simulink model "MMC_driven_PMSM_ideal"  (R2025b)
settings: Solver=FixedStepDiscrete  StartTime=0.0  StopTime=7  FixedStep=Ts  RelTol=1e-3
values from neighbouring files (symbols this model uses):
  Goff = 1e-06    [initParams.mat]
  Ron = 1e-06    [initParams.mat]
  Ts = 5e-05    [initParams.mat]
  Vcell = 1000    [initParams.mat]
undefined symbols (not defined in the file or in its folder): DiscIntNeverNeededParam
libraries: ee_lib_for_power_systems x50, fl_lib x48, nesl_utility x3, eeTransforms x2, ee_lib x2, simulink x1
(part 1 of 2)
settings Model: SimulationMode=accelerator  Creator=gdudgeon  LastModifiedBy=gdudgeon
settings SolverCC: AlgebraicLoopSolver=TrustRegion
settings DebuggingCC: UnconnectedInputMsg=warning  UnconnectedOutputMsg=warning  UnconnectedLineMsg=warning
settings ModelReferenceCC: EnableRefExpFcnMdlSchedulingChecks=on
settings RTWCC: GPUComputeCapability=3.5

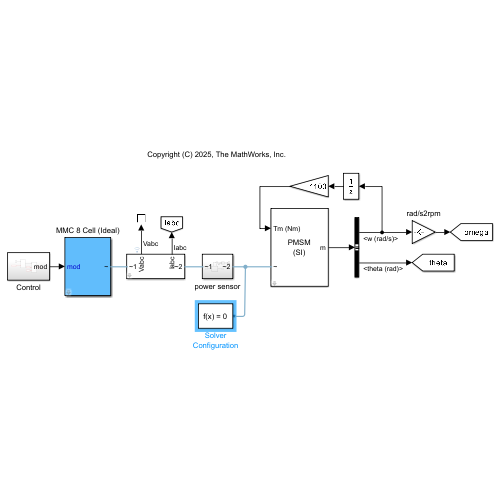
[thumbnail: Simulink's stored preview of the top-level diagram]
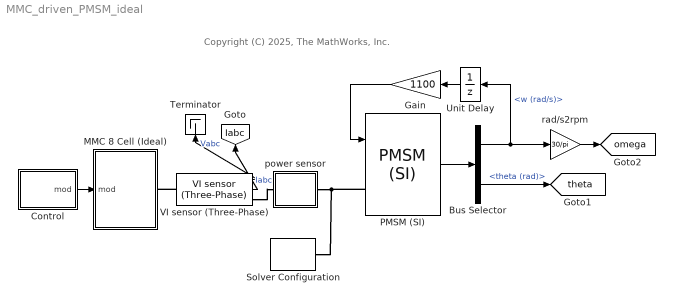
== system MMC_driven_PMSM_ideal ==
  note: Copyright (C) 2025, The MathWorks, Inc.
  Bus Selector : BusSelector  OutputSignals=w (rad/s),theta (rad)
  Control : Subsystem
  Gain : Gain  Gain=1100
  MMC 8 Cell (Ideal) : Subsystem  mask{Vcell=Vcell, freq=1000, no_cells=8}
      mask prompts: Vcell "Cell voltage (V)"; freq "Carrier frequency (Hz)"; no_cells "Number of cells"
  PMSM (SI) : ee_lib_for_power_systems/Electromechanical Machines/PMSM (SI)  run_time=on  p=1  flux_linkage=21  Ld=0.0005  Lq=0.0005  Rs=0.01  J=10  D=0
      settings: SourceProductName=Support Library for Power Systems
  Solver Configuration : nesl_utility/Solver Configuration  PhysicalDomain=network_engine_domain  SubClassName=solver  LeftPortType=input  RightPortType=generic  Tones=[]  Harmonics=[]  SimulateNoise=off  Profile=off  UseLocalSampling=off  EnableSwitchedLinearOptims=on  FrequencyDomain=off  UseCCode=off  RelTol=0.001  AbsTol=1e-06  MinStep=1e-09  ToWorkspace=off  RevertToSquareIcSolve=off  NumHomotopyIterations=100  PhasorMode=off  PhasorModeNumHarmonics=1  ConsistencySolver=NEWTON_FTOL  IndexReductionMethod=None  DoDC=off  ResidualTolerance=1e-09  ConsistencyTolSource=GLOBAL  ConsistencyAbsTol=0.001  ConsistencyRelTol=0.001  ConsistencyTolFactor=0.001  UseLocalSolver=on  LocalSolverChoice=NE_BACKWARD_EULER_ADVANCER  ResolveIndetEquations=off  FunctionEvalNumThread=1  LocalSolverSampleTime=TsELEC  DoFixedCost=on  MaxNonlinIter=1  MaxModeIter=2  ComputeImpulses=off  ImpulseIterations=2  LinearAlgebra=auto  LinearAlgebraNumThread=0  EquationFormulation=NE_TIME_EF  DelaysMemoryBudget=1024  AutomaticFiltering=off  FilteringTimeConstant=0.001  PartitionStorageMethod=AS_NEEDED  PartitionMemoryBudget=1024  PartitionMethod=ROBUST  MultibodyUseLocalSolver=off  MultibodyLocalSolverChoice=ODE1  MultibodyLocalSolverSampleTime=0.001
  Terminator : Terminator
  Unit Delay : UnitDelay  SampleTime=-1  HasFrameUpgradeWarning=on
  VI sensor (Three-Phase) : ee_lib_for_power_systems/Sense and Measure/VI sensor (Three-Phase)  volt_meas=Line-to-Line (Line Voltage)  meas_units=SI  Vnom=24e3  Pnom=100e6
      settings: SourceProductName=Support Library for Power Systems
  power sensor : Subsystem
  rad/s2rpm : Gain  Gain=30/pi
  tag scope: Iabc=global, omega=global, theta=global
  wires:
  Control/1(mod) -> MMC 8 Cell (Ideal)/1(mod)
  VI sensor (Three-Phase)/1 -> Terminator/1  "Vabc"
  VI sensor (Three-Phase)/2 -> [Iabc]  "Iabc"
  PMSM (SI)/1 -> Bus Selector/1
  Bus Selector/2 -> [theta]  "<theta (rad)>"
  Bus Selector/1 -> Unit Delay/1, rad/s2rpm/1  "<w (rad/s)>"
  Gain/1 -> PMSM (SI)/1
  Unit Delay/1 -> Gain/1
  rad/s2rpm/1 -> [omega]
  connections:
  VI sensor (Three-Phase)/RConn1 -- power sensor/LConn1
  VI sensor (Three-Phase)/LConn1 -- MMC 8 Cell (Ideal)/RConn1
  power sensor/RConn1 -- PMSM (SI)/LConn1 -- Solver Configuration/RConn1

== system MMC_driven_PMSM_ideal/Control ==
  Dead Zone : DeadZone  LowerValue=-0.001  UpperValue=0.001
  Speed Control : Subsystem
  Speed Reference (RPM) : simulink/Sources/Repeating Sequence Interpolated  OutValues=[0 0 1 1]*1800  TimeValues=[0 1 6 15]  LookUpMeth=Interpolation-Use End Values  tsamp=TsELEC  OutMin=[]  OutMax=[]  OutDataTypeStr=double  OutputDataTypeScalingMode=double  OutDataType=fixdt(0,8)  OutScaling=2^-10
  Torque Control : Subsystem
  Unit Delay1 : UnitDelay  SampleTime=Ts  HasFrameUpgradeWarning=on
  mod : Outport
  wires:
  Unit Delay1/1 -> Dead Zone/1
  Speed Reference (RPM)/1 -> Speed Control/1(Speed_Ref)  "omega_ref"
  Torque Control/1(mod) -> Unit Delay1/1
  [omega] -> Speed Control/2(Speed_Meas)  "omega"
  Speed Control/1(IdqRef) -> Torque Control/1(Idq_ref)
  [Iabc] -> Torque Control/2(Iabc_meas)
  [theta] -> Torque Control/3(theta)
  Dead Zone/1 -> mod/1

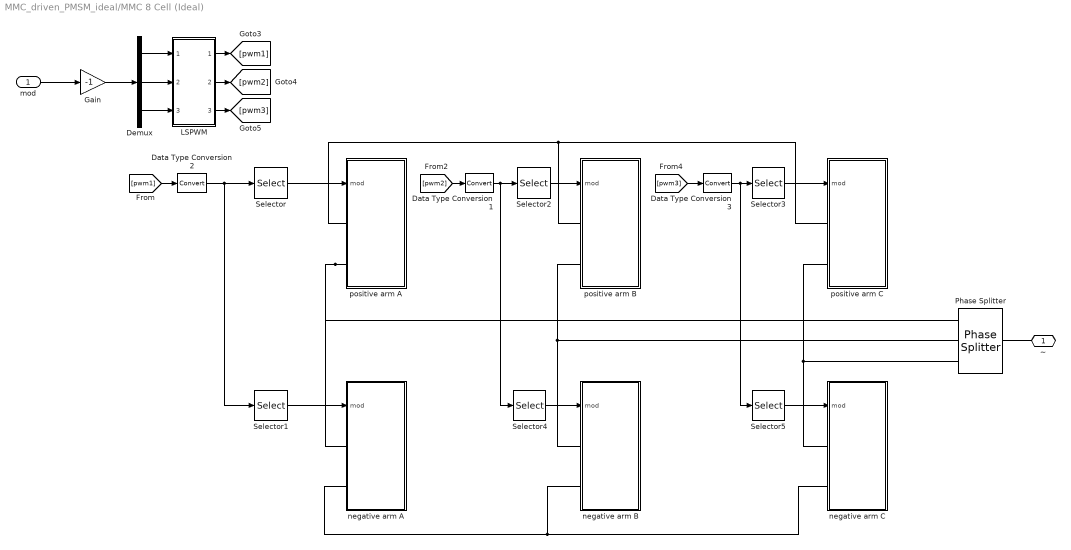
== system MMC_driven_PMSM_ideal/MMC 8 Cell (Ideal) ==
  mod : Inport
  Data Type Conversion1 : DataTypeConversion  SaturateOnIntegerOverflow=off  RndMeth=Floor
  Data Type Conversion2 : DataTypeConversion  SaturateOnIntegerOverflow=off  RndMeth=Floor
  Data Type Conversion3 : DataTypeConversion  SaturateOnIntegerOverflow=off  RndMeth=Floor
  Demux : Demux  Outputs=3
  Gain : Gain  Gain=-1
  LSPWM : Subsystem  mask{no_cells=no_cells, freq=freq}
      mask prompts: no_cells "Number of cells"; freq "Carrier frequency (Hz)"
  Phase Splitter : ee_lib/Connectors & References/Phase Splitter
  Selector : Selector  InputPortWidth=no_cells*4  IndexOptions=Index vector (dialog)  Indices=[1:(no_cells) (no_cells*2+1):no_cells*3]  OutputSizes=1
  Selector1 : Selector  InputPortWidth=no_cells*4  IndexOptions=Index vector (dialog)  Indices=[(no_cells)+(1:no_cells) (no_cells*3)+(1:no_cells)]  OutputSizes=1
  Selector2 : Selector  InputPortWidth=no_cells*4  IndexOptions=Index vector (dialog)  Indices=[1:(no_cells) (no_cells*2+1):no_cells*3]  OutputSizes=1
  Selector3 : Selector  InputPortWidth=no_cells*4  IndexOptions=Index vector (dialog)  Indices=[1:(no_cells) (no_cells*2+1):no_cells*3]  OutputSizes=1
  Selector4 : Selector  InputPortWidth=no_cells*4  IndexOptions=Index vector (dialog)  Indices=[(no_cells)+(1:no_cells) (no_cells*3)+(1:no_cells)]  OutputSizes=1
  Selector5 : Selector  InputPortWidth=no_cells*4  IndexOptions=Index vector (dialog)  Indices=[(no_cells)+(1:no_cells) (no_cells*3)+(1:no_cells)]  OutputSizes=1
  negative arm A : Subsystem  mask{Vcell=Vcell, no_cells=no_cells, Ron=Ron, Goff=Goff}
      mask prompts: Vcell "Cell Voltage (V)"; no_cells "Number of cells"; Ron "Ron (Ohm)"; Goff "Goff (1/Ohm)"
      mask init:
      | h = gcbh;
      | 
      | hr = find_system(h,'LookUnderMasks','All','RegExp','on','Name','rmod');
      | hs = find_system(h,'LookUnderMasks','All','RegExp','on','Name','smod');
      | 
      | for l = 1:numel(hr)
      |     
      |     nr = get(hr(l),'name');
      |     ns = get(hs(l),'name');
      |     
      |     set(hr(l),'GotoTag',nr(2:end));
      |     set(hs(l),'GotoTag',nr(2:end));
      |     
      | end
      |     
      | rr = zeros(1,no_cells*2);
      | rr(1:2:end) = 1:no_cells;
      | rr(2:2:end) = (no_cells+1):2*no_cells;
  negative arm B : Subsystem  mask{Vcell=Vcell, no_cells=no_cells, Ron=Ron, Goff=Goff}
      mask prompts: Vcell "Cell Voltage (V)"; no_cells "Number of cells"; Ron "Ron (Ohm)"; Goff "Goff (1/Ohm)"
      mask init: same as MMC_driven_PMSM_ideal/MMC 8 Cell (Ideal)/negative arm A
  negative arm C : Subsystem  mask{Vcell=Vcell, no_cells=no_cells, Ron=Ron, Goff=Goff}
      mask prompts: Vcell "Cell Voltage (V)"; no_cells "Number of cells"; Ron "Ron (Ohm)"; Goff "Goff (1/Ohm)"
      mask init: same as MMC_driven_PMSM_ideal/MMC 8 Cell (Ideal)/negative arm A
  positive arm A : Subsystem  mask{Vcell=Vcell, no_cells=no_cells, Ron=Ron, Goff=Goff}
      mask prompts: Vcell "Cell Voltage (V)"; no_cells "Number of cells"; Ron "Ron (Ohm)"; Goff "Goff (1/Ohm)"
      mask init: same as MMC_driven_PMSM_ideal/MMC 8 Cell (Ideal)/negative arm A
  positive arm B : Subsystem  mask{Vcell=Vcell, no_cells=no_cells, Ron=Ron, Goff=Goff}
      mask prompts: Vcell "Cell Voltage (V)"; no_cells "Number of cells"; Ron "Ron (Ohm)"; Goff "Goff (1/Ohm)"
      mask init: same as MMC_driven_PMSM_ideal/MMC 8 Cell (Ideal)/negative arm A
  positive arm C : Subsystem  mask{Vcell=Vcell, no_cells=no_cells, Ron=Ron, Goff=Goff}
      mask prompts: Vcell "Cell Voltage (V)"; no_cells "Number of cells"; Ron "Ron (Ohm)"; Goff "Goff (1/Ohm)"
      mask init: same as MMC_driven_PMSM_ideal/MMC 8 Cell (Ideal)/negative arm A
  ~ : PMIOPort  Side=Right
  wires:
  Gain/1 -> Demux/1
  Selector5/1 -> negative arm C/1(mod)
  Selector3/1 -> positive arm C/1(mod)
  Selector4/1 -> negative arm B/1(mod)
  Selector2/1 -> positive arm B/1(mod)
  Selector/1 -> positive arm A/1(mod)
  LSPWM/3("      ") -> [pwm3]
  LSPWM/2("       ") -> [pwm2]
  LSPWM/1(" ") -> [pwm1]
  [pwm3] -> Data Type Conversion3/1
  [pwm2] -> Data Type Conversion1/1
  [pwm1] -> Data Type Conversion2/1
  Demux/3 -> LSPWM/3("     ")
  Demux/2 -> LSPWM/2("   ")
  Demux/1 -> LSPWM/1("  ")
  mod/1 -> Gain/1
  Data Type Conversion2/1 -> Selector1/1, Selector/1
  Data Type Conversion3/1 -> Selector5/1, Selector3/1
  Data Type Conversion1/1 -> Selector2/1, Selector4/1
  Selector1/1 -> negative arm A/1(mod)
  connections:
  Phase Splitter/RConn2 -- negative arm B/LConn1 -- positive arm B/LConn2
  positive arm A/LConn2 -- negative arm A/LConn1 -- Phase Splitter/RConn1
  Phase Splitter/RConn3 -- positive arm C/LConn2 -- negative arm C/LConn1
  positive arm A/LConn1 -- positive arm C/LConn1 -- positive arm B/LConn1
  negative arm A/LConn2 -- negative arm C/LConn2 -- negative arm B/LConn2
  ~/RConn1 -- Phase Splitter/LConn1

== system MMC_driven_PMSM_ideal/power sensor ==
  PS-Simulink Converter : nesl_utility/PS-Simulink Converter  PhysicalDomain=network_engine_domain  SubClassName=ps_output  LeftPortType=input  RightPortType=output  PseudoPeriodic=off  Frequencies=[]  VectorFormat=inherit  Unit=inherit  AffineConversion=off
  PS-Simulink Converter1 : nesl_utility/PS-Simulink Converter  PhysicalDomain=network_engine_domain  SubClassName=ps_output  LeftPortType=input  RightPortType=output  PseudoPeriodic=off  Frequencies=[]  VectorFormat=inherit  Unit=inherit  AffineConversion=off
  Power Sensor (Three-Phase) : ee_lib/Sensors & Transducers/Power Sensor (Three-Phase)  load_type=ee.enum.passive.type_balanced.balanced  f0=60 Hz
      settings: InternalSimscapePortConfiguration="{\"Bottom\":[],\"Left\":[{\"id\":\"N1\",\"label\":\"~1\",\"type\":\"foundation.electrical.three_phase\"}],\"Right\":[{\"id\":\"N2\",\"label\":\"~2\",\"type\":\"foundation.electrical.three_phase\"}],\"Top\":[{\"id\":\"Pm\",\"label\":\"P\",\"type\":\"output\"},{\"id\":\"Qm\",\"label\":\"Q\",\"type\":\"output\"}]}"
  Subsystem1 : Subsystem
  Subsystem2 : Subsystem
  Terminator : Terminator
  Terminator1 : Terminator
  ~1 : PMIOPort  Side=Left
  ~2 : PMIOPort  Port=2  Side=Right
  wires:
  PS-Simulink Converter/1 -> Subsystem1/1(In1)
  PS-Simulink Converter1/1 -> Subsystem2/1(In1)
  Subsystem2/1(Out1) -> Terminator1/1  "Q"
  Subsystem1/1(Out1) -> Terminator/1  "P"
  connections:
  Power Sensor (Three-Phase)/LConn2 -- PS-Simulink Converter/LConn1
  Power Sensor (Three-Phase)/RConn1 -- ~2/RConn1
  Power Sensor (Three-Phase)/LConn1 -- ~1/RConn1
  Power Sensor (Three-Phase)/LConn3 -- PS-Simulink Converter1/LConn1

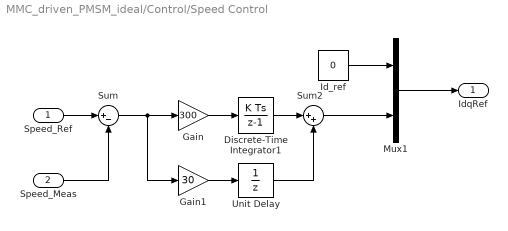
== system MMC_driven_PMSM_ideal/Control/Speed Control ==
  Speed_Ref : Inport
  Speed_Meas : Inport  Port=2
  Discrete-Time Integrator1 : DiscreteIntegrator  SampleTime=Ts  ICPrevOutput=DiscIntNeverNeededParam  ICPrevScaledInput=DiscIntNeverNeededParam
  Gain : Gain  Gain=300
  Gain1 : Gain  Gain=30
  Id_ref : Constant  Value=0  OutDataTypeStr=Inherit: Inherit via back propagation  SampleTime=Ts
  Mux1 : Mux  Inputs=2
  Sum : Sum  Inputs=|+-
  Sum2 : Sum  Inputs=|++
  Unit Delay : UnitDelay  SampleTime=Ts  HasFrameUpgradeWarning=on
  IdqRef : Outport  VectorParamsAs1DForOutWhenUnconnected=off
  wires:
  Sum2/1 -> Mux1/2
  Id_ref/1 -> Mux1/1
  Speed_Ref/1 -> Sum/1
  Speed_Meas/1 -> Sum/2
  Mux1/1 -> IdqRef/1
  Gain/1 -> Discrete-Time Integrator1/1
  Sum/1 -> Gain1/1, Gain/1
  Unit Delay/1 -> Sum2/2
  Gain1/1 -> Unit Delay/1
  Discrete-Time Integrator1/1 -> Sum2/1

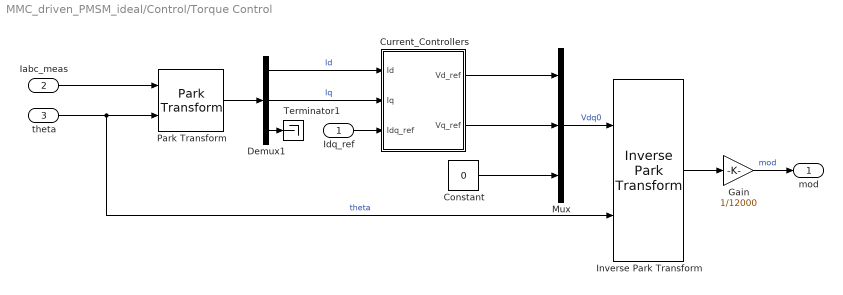
== system MMC_driven_PMSM_ideal/Control/Torque Control ==
  Idq_ref : Inport
  Iabc_meas : Inport  Port=2
  theta : Inport  Port=3
  Constant : Constant  Value=0  SampleTime=Ts
  Current_Controllers : Subsystem
  Demux1 : Demux  Outputs=3
  Gain : Gain  Gain=1/12000
  Inverse Park Transform : eeTransforms/Inverse Park Transform  AxisAlignment=Q-axis  PowerInvariant=off
  Mux : Mux  Inputs=3
  Park Transform : eeTransforms/Park Transform  AxisAlignment=Q-axis  PowerInvariant=off
      settings: LibrarySourceBlock=|
      | ee_sl_lib/Mathematical
      | Transforms/Park Transform
  Terminator1 : Terminator
  mod : Outport  VectorParamsAs1DForOutWhenUnconnected=off
  wires:
  Current_Controllers/1(Vd_ref) -> Mux/1
  Gain/1 -> mod/1  "mod"
  Idq_ref/1 -> Current_Controllers/3(Idq_ref)
  Inverse Park Transform/1 -> Gain/1
  Park Transform/1 -> Demux1/1
  Constant/1 -> Mux/3
  Demux1/2 -> Current_Controllers/2(Iq)  "Iq"
  Current_Controllers/2(Vq_ref) -> Mux/2
  Demux1/3 -> Terminator1/1
  Mux/1 -> Inverse Park Transform/1  "Vdq0"
  theta/1 -> Inverse Park Transform/2, Park Transform/2  "theta"
  Demux1/1 -> Current_Controllers/1(Id)  "Id"
  Iabc_meas/1 -> Park Transform/1

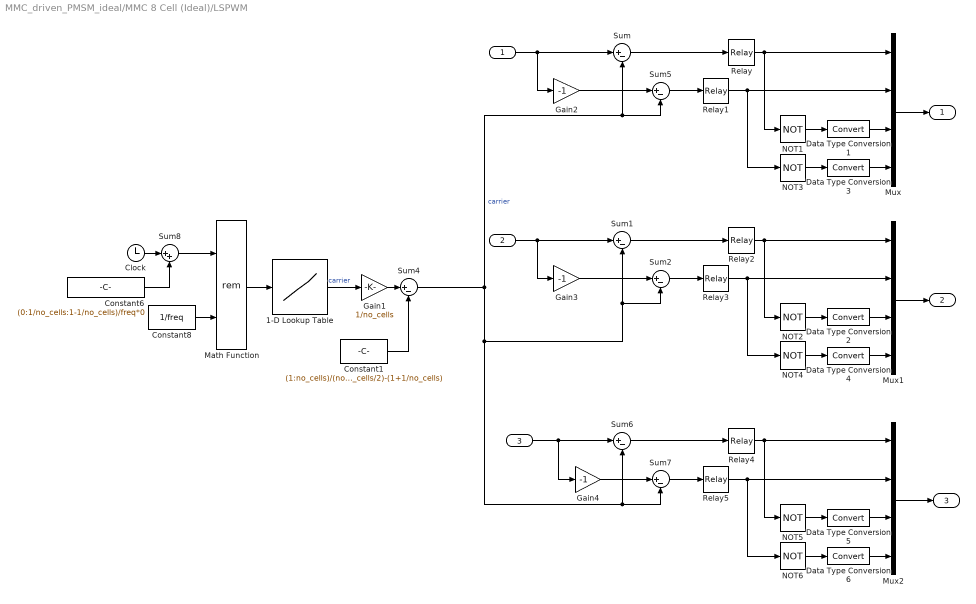
== system MMC_driven_PMSM_ideal/MMC 8 Cell (Ideal)/LSPWM ==
  "  " : Inport
  "   " : Inport  Port=2
  "     " : Inport  Port=3
  1-D Lookup Table : Lookup_n-D  NumberOfTableDimensions=1  BreakpointsForDimension1=[0 1 2 3 4]/4/freq  Table=[0 1 0 -1 0]  RndMeth=Simplest
  Clock : Clock
  Constant1 : Constant  DisableCoverage=on  Value=(1:no_cells)/(no_cells/2)-(1+1/no_cells)  SampleTime=0
  Constant6 : Constant  Value=(0:1/no_cells:1-1/no_cells)/freq*0  SampleTime=0
  Constant8 : Constant  DisableCoverage=on  Value=1/freq  SampleTime=0
  Data Type Conversion{1..6} (6 alike) : DataTypeConversion  SaturateOnIntegerOverflow=off  RndMeth=Floor
  Gain1 : Gain  Gain=1/no_cells
  Gain2 : Gain  Gain=-1
  Gain3 : Gain  Gain=-1
  Gain4 : Gain  Gain=-1
  Math Function : Math  DisableCoverage=on  Operator=rem  SignedPower=on
  Mux : Mux
  Mux1 : Mux
  Mux2 : Mux
  NOT{1..6} (6 alike) : Logic  Operator=NOT  IconShape=distinctive  AllPortsSameDT=off  OutDataTypeStr=boolean
  Relay{,1..5} (6 alike) : Relay
  Sum{,1..2,4..7} (7 alike) : Sum  Inputs=|+-
  Sum8 : Sum  Inputs=|++
  " " : Outport  VectorParamsAs1DForOutWhenUnconnected=off
  "       " : Outport  Port=2  VectorParamsAs1DForOutWhenUnconnected=off
  "      " : Outport  Port=3  VectorParamsAs1DForOutWhenUnconnected=off
  wires:
  Sum4/1 -> Sum/2, Sum5/2, Sum6/2, Sum7/2, Sum2/2, Sum1/2  "carrier"
  Relay5/1 -> Mux2/2, NOT6/1
  Sum7/1 -> Relay5/1
  Gain4/1 -> Sum7/1
  Data Type Conversion6/1 -> Mux2/4
  NOT6/1 -> Data Type Conversion6/1
  Data Type Conversion5/1 -> Mux2/3
  "     "/1 -> Gain4/1, Sum6/1
  Sum6/1 -> Relay4/1
  Relay4/1 -> Mux2/1, NOT5/1
  NOT5/1 -> Data Type Conversion5/1
  Mux2/1 -> "      "/1
  Mux1/1 -> "       "/1
  NOT2/1 -> Data Type Conversion2/1
  Relay2/1 -> NOT2/1, Mux1/1
  Sum1/1 -> Relay2/1
  "   "/1 -> Sum1/1, Gain3/1
  Data Type Conversion2/1 -> Mux1/3
  NOT4/1 -> Data Type Conversion4/1
  Data Type Conversion4/1 -> Mux1/4
  Gain3/1 -> Sum2/1
  Sum2/1 -> Relay3/1
  Relay3/1 -> NOT4/1, Mux1/2
  Relay1/1 -> Mux/2, NOT3/1
  Sum5/1 -> Relay1/1
  Gain2/1 -> Sum5/1
  Data Type Conversion3/1 -> Mux/4
  NOT3/1 -> Data Type Conversion3/1
  Data Type Conversion1/1 -> Mux/3
  Gain1/1 -> Sum4/1
  Constant1/1 -> Sum4/2
  1-D Lookup Table/1 -> Gain1/1  "carrier"
  Mux/1 -> " "/1
  Sum8/1 -> Math Function/1
  Math Function/1 -> 1-D Lookup Table/1
  Constant8/1 -> Math Function/2
  Constant6/1 -> Sum8/2
  Clock/1 -> Sum8/1
  "  "/1 -> Gain2/1, Sum/1
  Sum/1 -> Relay/1
  Relay/1 -> Mux/1, NOT1/1
  NOT1/1 -> Data Type Conversion1/1

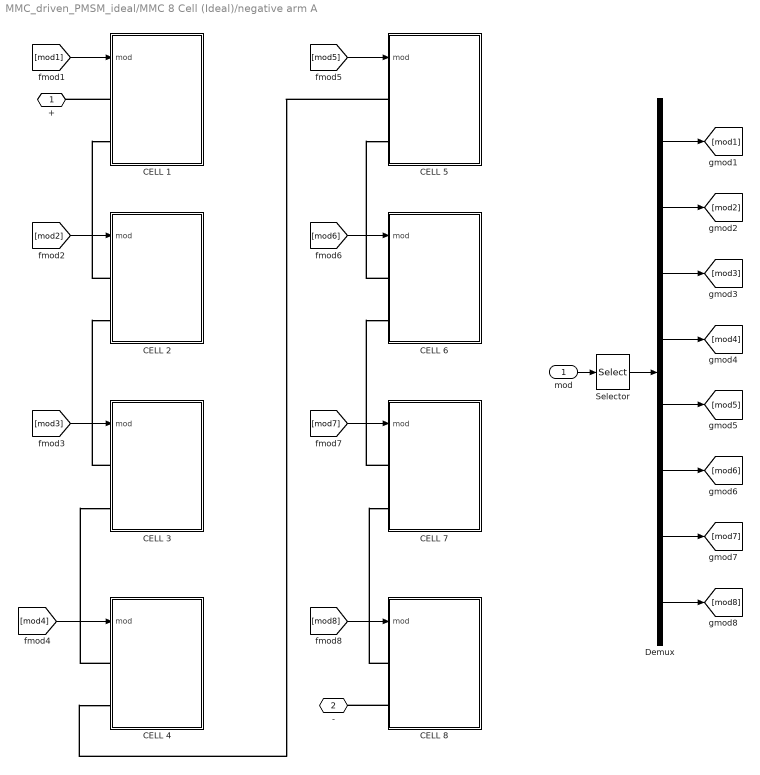
== system MMC_driven_PMSM_ideal/MMC 8 Cell (Ideal)/negative arm A ==
  mod : Inport
  CELL 1 : Subsystem
  CELL 2 : Subsystem
  CELL 3 : Subsystem
  CELL 4 : Subsystem
  CELL 5 : Subsystem
  CELL 6 : Subsystem
  CELL 7 : Subsystem
  CELL 8 : Subsystem
  Demux : Demux  Outputs=8
  Selector : Selector  InputPortWidth=2*no_cells  IndexOptions=Index vector (dialog)  Indices=rr  OutputSizes=1
  "+ " : PMIOPort  Side=Left
  "- " : PMIOPort  Port=2  Side=Left
  wires:
  Demux/8 -> [mod8]
  Demux/7 -> [mod7]
  Demux/6 -> [mod6]
  Demux/5 -> [mod5]
  Demux/4 -> [mod4]
  [mod4] -> CELL 4/1(mod)
  Demux/3 -> [mod3]
  [mod3] -> CELL 3/1(mod)
  Demux/2 -> [mod2]
  [mod2] -> CELL 2/1(mod)
  Demux/1 -> [mod1]
  [mod1] -> CELL 1/1(mod)
  mod/1 -> Selector/1
  Selector/1 -> Demux/1
  [mod5] -> CELL 5/1(mod)
  [mod6] -> CELL 6/1(mod)
  [mod7] -> CELL 7/1(mod)
  [mod8] -> CELL 8/1(mod)
  connections:
  CELL 1/LConn1 -- "+ "/RConn1
  CELL 5/LConn1 -- CELL 4/LConn2
  CELL 4/LConn1 -- CELL 3/LConn2
  CELL 3/LConn1 -- CELL 2/LConn2
  CELL 2/LConn1 -- CELL 1/LConn2
  CELL 6/LConn1 -- CELL 5/LConn2
  CELL 7/LConn1 -- CELL 6/LConn2
  CELL 8/LConn1 -- CELL 7/LConn2
  CELL 8/LConn2 -- "- "/RConn1

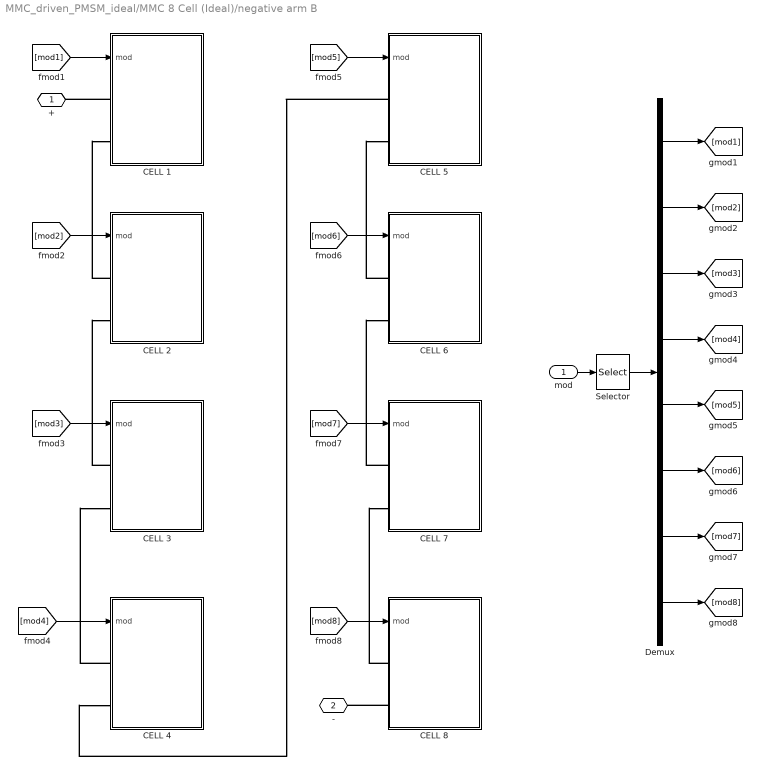
== system MMC_driven_PMSM_ideal/MMC 8 Cell (Ideal)/negative arm B ==
  mod : Inport
  CELL 1 : Subsystem
  CELL 2 : Subsystem
  CELL 3 : Subsystem
  CELL 4 : Subsystem
  CELL 5 : Subsystem
  CELL 6 : Subsystem
  CELL 7 : Subsystem
  CELL 8 : Subsystem
  Demux : Demux  Outputs=8
  Selector : Selector  InputPortWidth=2*no_cells  IndexOptions=Index vector (dialog)  Indices=rr  OutputSizes=1
  "+ " : PMIOPort  Side=Left
  "- " : PMIOPort  Port=2  Side=Left
  wires:
  [mod8] -> CELL 8/1(mod)
  [mod7] -> CELL 7/1(mod)
  [mod6] -> CELL 6/1(mod)
  [mod5] -> CELL 5/1(mod)
  Selector/1 -> Demux/1
  mod/1 -> Selector/1
  [mod1] -> CELL 1/1(mod)
  Demux/1 -> [mod1]
  [mod2] -> CELL 2/1(mod)
  Demux/2 -> [mod2]
  [mod3] -> CELL 3/1(mod)
  Demux/3 -> [mod3]
  [mod4] -> CELL 4/1(mod)
  Demux/4 -> [mod4]
  Demux/5 -> [mod5]
  Demux/6 -> [mod6]
  Demux/7 -> [mod7]
  Demux/8 -> [mod8]
  connections:
  CELL 8/LConn2 -- "- "/RConn1
  CELL 8/LConn1 -- CELL 7/LConn2
  CELL 7/LConn1 -- CELL 6/LConn2
  CELL 6/LConn1 -- CELL 5/LConn2
  CELL 2/LConn1 -- CELL 1/LConn2
  CELL 3/LConn1 -- CELL 2/LConn2
  CELL 4/LConn1 -- CELL 3/LConn2
  CELL 5/LConn1 -- CELL 4/LConn2
  CELL 1/LConn1 -- "+ "/RConn1

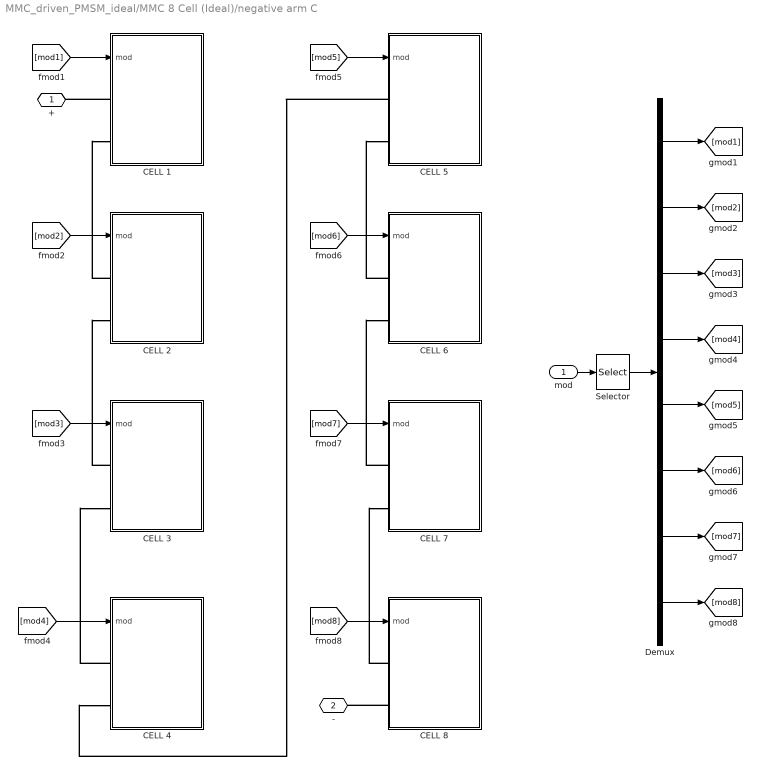
== system MMC_driven_PMSM_ideal/MMC 8 Cell (Ideal)/negative arm C ==
  mod : Inport
  CELL 1 : Subsystem
  CELL 2 : Subsystem
  CELL 3 : Subsystem
  CELL 4 : Subsystem
  CELL 5 : Subsystem
  CELL 6 : Subsystem
  CELL 7 : Subsystem
  CELL 8 : Subsystem
  Demux : Demux  Outputs=8
  Selector : Selector  InputPortWidth=2*no_cells  IndexOptions=Index vector (dialog)  Indices=rr  OutputSizes=1
  "+ " : PMIOPort  Side=Left
  "- " : PMIOPort  Port=2  Side=Left
  wires:
  Demux/8 -> [mod8]
  Demux/7 -> [mod7]
  Demux/6 -> [mod6]
  Demux/5 -> [mod5]
  Demux/4 -> [mod4]
  [mod4] -> CELL 4/1(mod)
  Demux/3 -> [mod3]
  [mod3] -> CELL 3/1(mod)
  Demux/2 -> [mod2]
  [mod2] -> CELL 2/1(mod)
  Demux/1 -> [mod1]
  [mod1] -> CELL 1/1(mod)
  mod/1 -> Selector/1
  Selector/1 -> Demux/1
  [mod5] -> CELL 5/1(mod)
  [mod6] -> CELL 6/1(mod)
  [mod7] -> CELL 7/1(mod)
  [mod8] -> CELL 8/1(mod)
  connections:
  CELL 1/LConn1 -- "+ "/RConn1
  CELL 5/LConn1 -- CELL 4/LConn2
  CELL 4/LConn1 -- CELL 3/LConn2
  CELL 3/LConn1 -- CELL 2/LConn2
  CELL 2/LConn1 -- CELL 1/LConn2
  CELL 6/LConn1 -- CELL 5/LConn2
  CELL 7/LConn1 -- CELL 6/LConn2
  CELL 8/LConn1 -- CELL 7/LConn2
  CELL 8/LConn2 -- "- "/RConn1

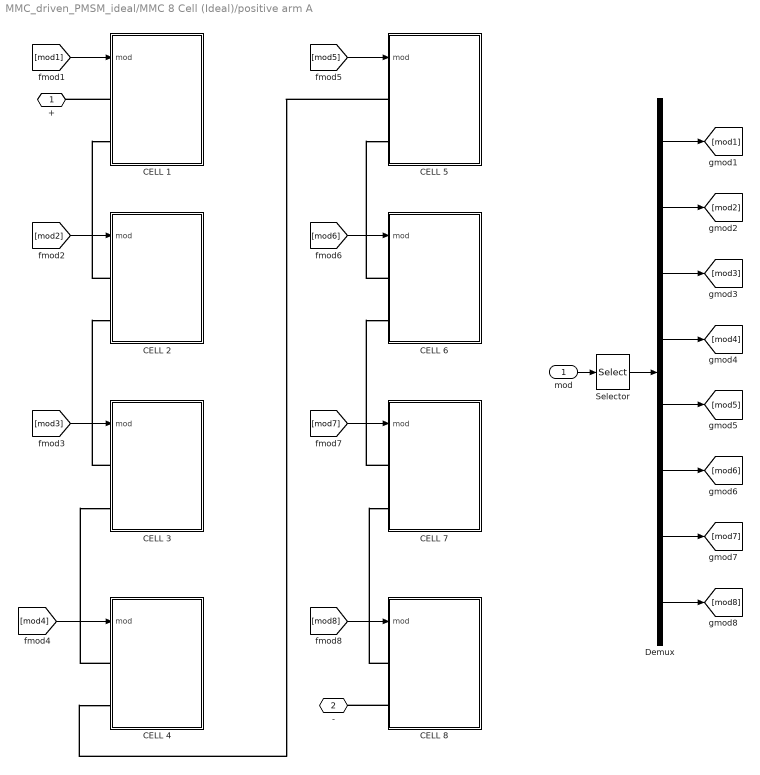
== system MMC_driven_PMSM_ideal/MMC 8 Cell (Ideal)/positive arm A ==
  mod : Inport
  CELL 1 : Subsystem
  CELL 2 : Subsystem
  CELL 3 : Subsystem
  CELL 4 : Subsystem
  CELL 5 : Subsystem
  CELL 6 : Subsystem
  CELL 7 : Subsystem
  CELL 8 : Subsystem
  Demux : Demux  Outputs=8
  Selector : Selector  InputPortWidth=2*no_cells  IndexOptions=Index vector (dialog)  Indices=rr  OutputSizes=1
  "+ " : PMIOPort  Side=Left
  "- " : PMIOPort  Port=2  Side=Left
  wires:
  [mod8] -> CELL 8/1(mod)
  [mod7] -> CELL 7/1(mod)
  [mod6] -> CELL 6/1(mod)
  [mod5] -> CELL 5/1(mod)
  Selector/1 -> Demux/1
  mod/1 -> Selector/1
  [mod1] -> CELL 1/1(mod)
  Demux/1 -> [mod1]
  [mod2] -> CELL 2/1(mod)
  Demux/2 -> [mod2]
  [mod3] -> CELL 3/1(mod)
  Demux/3 -> [mod3]
  [mod4] -> CELL 4/1(mod)
  Demux/4 -> [mod4]
  Demux/5 -> [mod5]
  Demux/6 -> [mod6]
  Demux/7 -> [mod7]
  Demux/8 -> [mod8]
  connections:
  CELL 8/LConn2 -- "- "/RConn1
  CELL 8/LConn1 -- CELL 7/LConn2
  CELL 7/LConn1 -- CELL 6/LConn2
  CELL 6/LConn1 -- CELL 5/LConn2
  CELL 2/LConn1 -- CELL 1/LConn2
  CELL 3/LConn1 -- CELL 2/LConn2
  CELL 4/LConn1 -- CELL 3/LConn2
  CELL 5/LConn1 -- CELL 4/LConn2
  CELL 1/LConn1 -- "+ "/RConn1

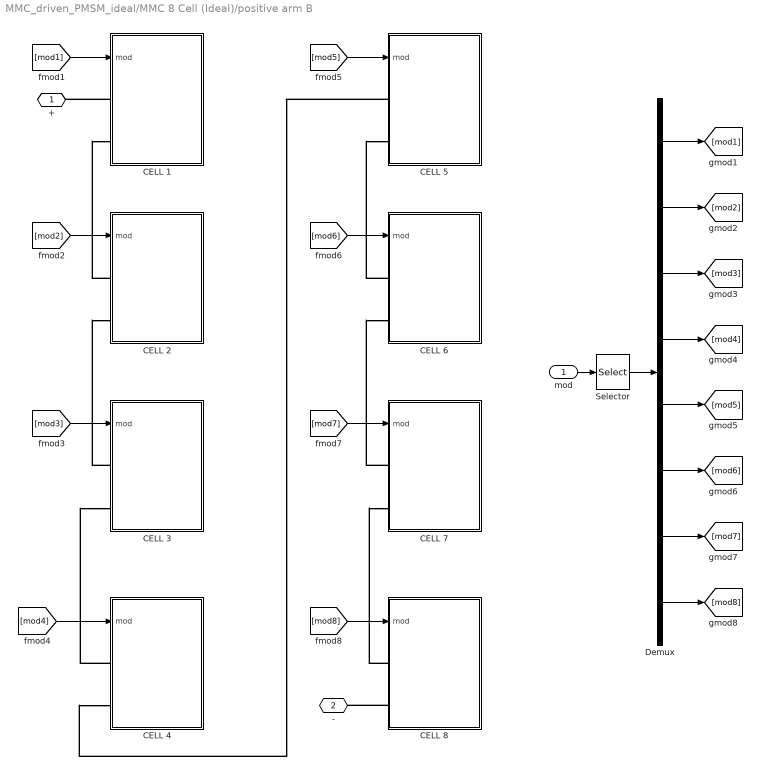
== system MMC_driven_PMSM_ideal/MMC 8 Cell (Ideal)/positive arm B ==
  mod : Inport
  CELL 1 : Subsystem
  CELL 2 : Subsystem
  CELL 3 : Subsystem
  CELL 4 : Subsystem
  CELL 5 : Subsystem
  CELL 6 : Subsystem
  CELL 7 : Subsystem
  CELL 8 : Subsystem
  Demux : Demux  Outputs=8
  Selector : Selector  InputPortWidth=2*no_cells  IndexOptions=Index vector (dialog)  Indices=rr  OutputSizes=1
  "+ " : PMIOPort  Side=Left
  "- " : PMIOPort  Port=2  Side=Left
  wires:
  Demux/8 -> [mod8]
  Demux/7 -> [mod7]
  Demux/6 -> [mod6]
  Demux/5 -> [mod5]
  Demux/4 -> [mod4]
  [mod4] -> CELL 4/1(mod)
  Demux/3 -> [mod3]
  [mod3] -> CELL 3/1(mod)
  Demux/2 -> [mod2]
  [mod2] -> CELL 2/1(mod)
  Demux/1 -> [mod1]
  [mod1] -> CELL 1/1(mod)
  mod/1 -> Selector/1
  Selector/1 -> Demux/1
  [mod5] -> CELL 5/1(mod)
  [mod6] -> CELL 6/1(mod)
  [mod7] -> CELL 7/1(mod)
  [mod8] -> CELL 8/1(mod)
  connections:
  CELL 1/LConn1 -- "+ "/RConn1
  CELL 5/LConn1 -- CELL 4/LConn2
  CELL 4/LConn1 -- CELL 3/LConn2
  CELL 3/LConn1 -- CELL 2/LConn2
  CELL 2/LConn1 -- CELL 1/LConn2
  CELL 6/LConn1 -- CELL 5/LConn2
  CELL 7/LConn1 -- CELL 6/LConn2
  CELL 8/LConn1 -- CELL 7/LConn2
  CELL 8/LConn2 -- "- "/RConn1

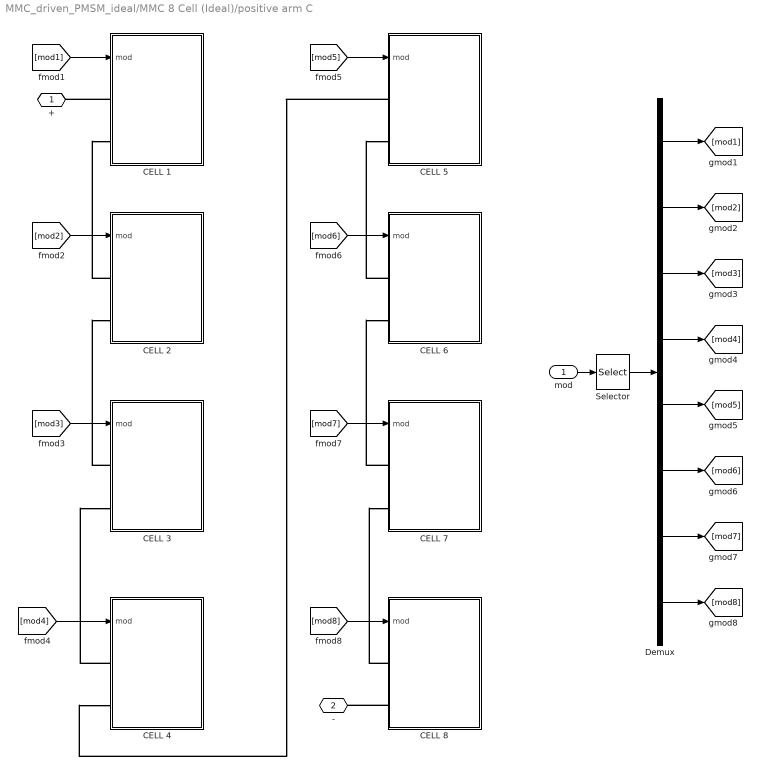
== system MMC_driven_PMSM_ideal/MMC 8 Cell (Ideal)/positive arm C ==
  mod : Inport
  CELL 1 : Subsystem
  CELL 2 : Subsystem
  CELL 3 : Subsystem
  CELL 4 : Subsystem
  CELL 5 : Subsystem
  CELL 6 : Subsystem
  CELL 7 : Subsystem
  CELL 8 : Subsystem
  Demux : Demux  Outputs=8
  Selector : Selector  InputPortWidth=2*no_cells  IndexOptions=Index vector (dialog)  Indices=rr  OutputSizes=1
  "+ " : PMIOPort  Side=Left
  "- " : PMIOPort  Port=2  Side=Left
  wires:
  [mod8] -> CELL 8/1(mod)
  [mod7] -> CELL 7/1(mod)
  [mod6] -> CELL 6/1(mod)
  [mod5] -> CELL 5/1(mod)
  Selector/1 -> Demux/1
  mod/1 -> Selector/1
  [mod1] -> CELL 1/1(mod)
  Demux/1 -> [mod1]
  [mod2] -> CELL 2/1(mod)
  Demux/2 -> [mod2]
  [mod3] -> CELL 3/1(mod)
  Demux/3 -> [mod3]
  [mod4] -> CELL 4/1(mod)
  Demux/4 -> [mod4]
  Demux/5 -> [mod5]
  Demux/6 -> [mod6]
  Demux/7 -> [mod7]
  Demux/8 -> [mod8]
  connections:
  CELL 8/LConn2 -- "- "/RConn1
  CELL 8/LConn1 -- CELL 7/LConn2
  CELL 7/LConn1 -- CELL 6/LConn2
  CELL 6/LConn1 -- CELL 5/LConn2
  CELL 2/LConn1 -- CELL 1/LConn2
  CELL 3/LConn1 -- CELL 2/LConn2
  CELL 4/LConn1 -- CELL 3/LConn2
  CELL 5/LConn1 -- CELL 4/LConn2
  CELL 1/LConn1 -- "+ "/RConn1

== system MMC_driven_PMSM_ideal/power sensor/Subsystem1 ==
  In1 : Inport
  Discrete-Time Integrator : DiscreteIntegrator  gainval=100  SampleTime=-1  ICPrevOutput=DiscIntNeverNeededParam  ICPrevScaledInput=DiscIntNeverNeededParam
  Sum : Sum  Inputs=|+-
  Out1 : Outport
  wires:
  Sum/1 -> Discrete-Time Integrator/1
  Discrete-Time Integrator/1 -> Out1/1, Sum/2
  In1/1 -> Sum/1

== system MMC_driven_PMSM_ideal/power sensor/Subsystem2 ==
  In1 : Inport
  Discrete-Time Integrator : DiscreteIntegrator  gainval=100  SampleTime=-1  ICPrevOutput=DiscIntNeverNeededParam  ICPrevScaledInput=DiscIntNeverNeededParam
  Sum : Sum  Inputs=|+-
  Out1 : Outport
  wires:
  In1/1 -> Sum/1
  Discrete-Time Integrator/1 -> Sum/2, Out1/1
  Sum/1 -> Discrete-Time Integrator/1

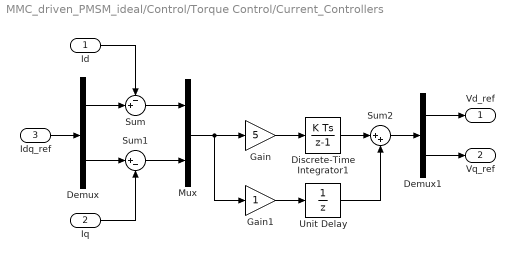
== system MMC_driven_PMSM_ideal/Control/Torque Control/Current_Controllers ==
  Id : Inport
  Iq : Inport  Port=2
  Idq_ref : Inport  Port=3
  Demux : Demux  Outputs=2
  Demux1 : Demux  Outputs=2
  Discrete-Time Integrator1 : DiscreteIntegrator  SampleTime=Ts  ICPrevOutput=DiscIntNeverNeededParam  ICPrevScaledInput=DiscIntNeverNeededParam
  Gain : Gain  Gain=5
  Gain1 : Gain
  Mux : Mux  Inputs=2
  Sum : Sum  Inputs=-+|
  Sum1 : Sum  Inputs=|+-
  Sum2 : Sum  Inputs=|++
  Unit Delay : UnitDelay  SampleTime=Ts  HasFrameUpgradeWarning=on
  Vd_ref : Outport  VectorParamsAs1DForOutWhenUnconnected=off
  Vq_ref : Outport  Port=2  VectorParamsAs1DForOutWhenUnconnected=off
  wires:
  Demux/2 -> Sum1/1
  Idq_ref/1 -> Demux/1
  Discrete-Time Integrator1/1 -> Sum2/1
  Unit Delay/1 -> Sum2/2
  Gain/1 -> Discrete-Time Integrator1/1
  Gain1/1 -> Unit Delay/1
  Sum2/1 -> Demux1/1
  Demux1/1 -> Vd_ref/1
  Demux1/2 -> Vq_ref/1
  Iq/1 -> Sum1/2
  Sum1/1 -> Mux/2
  Mux/1 -> Gain1/1, Gain/1
  Sum/1 -> Mux/1
  Demux/1 -> Sum/2
  Id/1 -> Sum/1

== system MMC_driven_PMSM_ideal/MMC 8 Cell (Ideal)/negative arm A/CELL 1 ==
  mod : Inport
  DC Voltage Source : fl_lib/Electrical/Electrical Sources/DC Voltage Source  v0=Vcell V
  Ideal Half-Bridge : ee_lib_for_power_systems/Power Converters/Ideal Half-Bridge  Vf=0.5  Ron=Ron  Goff=Goff  run_time=off
      settings: SourceProductName=Support Library for Power Systems
  + : PMIOPort  Side=Left
  - : PMIOPort  Port=2  Side=Left
  wires:
  mod/1 -> Ideal Half-Bridge/1
  connections:
  Ideal Half-Bridge/LConn1 -- +/RConn1
  Ideal Half-Bridge/RConn1 -- DC Voltage Source/LConn1
  Ideal Half-Bridge/RConn2 -- DC Voltage Source/RConn1 -- -/RConn1

== system MMC_driven_PMSM_ideal/MMC 8 Cell (Ideal)/negative arm A/CELL 2 ==
  mod : Inport
  DC Voltage Source : fl_lib/Electrical/Electrical Sources/DC Voltage Source  v0=Vcell V
  Ideal Half-Bridge : ee_lib_for_power_systems/Power Converters/Ideal Half-Bridge  Vf=0.5  Ron=Ron  Goff=Goff  run_time=off
      settings: SourceProductName=Support Library for Power Systems
  + : PMIOPort  Side=Left
  - : PMIOPort  Port=2  Side=Left
  wires:
  mod/1 -> Ideal Half-Bridge/1
  connections:
  -/RConn1 -- DC Voltage Source/RConn1 -- Ideal Half-Bridge/RConn2
  Ideal Half-Bridge/RConn1 -- DC Voltage Source/LConn1
  Ideal Half-Bridge/LConn1 -- +/RConn1

== system MMC_driven_PMSM_ideal/MMC 8 Cell (Ideal)/negative arm A/CELL 3 ==
  mod : Inport
  DC Voltage Source : fl_lib/Electrical/Electrical Sources/DC Voltage Source  v0=Vcell V
  Ideal Half-Bridge : ee_lib_for_power_systems/Power Converters/Ideal Half-Bridge  Vf=0.5  Ron=Ron  Goff=Goff  run_time=off
      settings: SourceProductName=Support Library for Power Systems
  + : PMIOPort  Side=Left
  - : PMIOPort  Port=2  Side=Left
  wires:
  mod/1 -> Ideal Half-Bridge/1
  connections:
  Ideal Half-Bridge/LConn1 -- +/RConn1
  Ideal Half-Bridge/RConn1 -- DC Voltage Source/LConn1
  Ideal Half-Bridge/RConn2 -- DC Voltage Source/RConn1 -- -/RConn1

== system MMC_driven_PMSM_ideal/MMC 8 Cell (Ideal)/negative arm A/CELL 4 ==
  mod : Inport
  DC Voltage Source : fl_lib/Electrical/Electrical Sources/DC Voltage Source  v0=Vcell V
  Ideal Half-Bridge : ee_lib_for_power_systems/Power Converters/Ideal Half-Bridge  Vf=0.5  Ron=Ron  Goff=Goff  run_time=off
      settings: SourceProductName=Support Library for Power Systems
  + : PMIOPort  Side=Left
  - : PMIOPort  Port=2  Side=Left
  wires:
  mod/1 -> Ideal Half-Bridge/1
  connections:
  -/RConn1 -- DC Voltage Source/RConn1 -- Ideal Half-Bridge/RConn2
  Ideal Half-Bridge/RConn1 -- DC Voltage Source/LConn1
  Ideal Half-Bridge/LConn1 -- +/RConn1

== system MMC_driven_PMSM_ideal/MMC 8 Cell (Ideal)/negative arm A/CELL 5 ==
  mod : Inport
  DC Voltage Source : fl_lib/Electrical/Electrical Sources/DC Voltage Source  v0=Vcell V
  Ideal Half-Bridge : ee_lib_for_power_systems/Power Converters/Ideal Half-Bridge  Vf=0.5  Ron=Ron  Goff=Goff  run_time=off
      settings: SourceProductName=Support Library for Power Systems
  + : PMIOPort  Side=Left
  - : PMIOPort  Port=2  Side=Left
  wires:
  mod/1 -> Ideal Half-Bridge/1
  connections:
  Ideal Half-Bridge/LConn1 -- +/RConn1
  Ideal Half-Bridge/RConn1 -- DC Voltage Source/LConn1
  Ideal Half-Bridge/RConn2 -- DC Voltage Source/RConn1 -- -/RConn1

== system MMC_driven_PMSM_ideal/MMC 8 Cell (Ideal)/negative arm A/CELL 6 ==
  mod : Inport
  DC Voltage Source : fl_lib/Electrical/Electrical Sources/DC Voltage Source  v0=Vcell V
  Ideal Half-Bridge : ee_lib_for_power_systems/Power Converters/Ideal Half-Bridge  Vf=0.5  Ron=Ron  Goff=Goff  run_time=off
      settings: SourceProductName=Support Library for Power Systems
  + : PMIOPort  Side=Left
  - : PMIOPort  Port=2  Side=Left
  wires:
  mod/1 -> Ideal Half-Bridge/1
  connections:
  -/RConn1 -- DC Voltage Source/RConn1 -- Ideal Half-Bridge/RConn2
  Ideal Half-Bridge/RConn1 -- DC Voltage Source/LConn1
  Ideal Half-Bridge/LConn1 -- +/RConn1

== system MMC_driven_PMSM_ideal/MMC 8 Cell (Ideal)/negative arm A/CELL 7 ==
  mod : Inport
  DC Voltage Source : fl_lib/Electrical/Electrical Sources/DC Voltage Source  v0=Vcell V
  Ideal Half-Bridge : ee_lib_for_power_systems/Power Converters/Ideal Half-Bridge  Vf=0.5  Ron=Ron  Goff=Goff  run_time=off
      settings: SourceProductName=Support Library for Power Systems
  + : PMIOPort  Side=Left
  - : PMIOPort  Port=2  Side=Left
  wires:
  mod/1 -> Ideal Half-Bridge/1
  connections:
  Ideal Half-Bridge/LConn1 -- +/RConn1
  Ideal Half-Bridge/RConn1 -- DC Voltage Source/LConn1
  Ideal Half-Bridge/RConn2 -- DC Voltage Source/RConn1 -- -/RConn1

== system MMC_driven_PMSM_ideal/MMC 8 Cell (Ideal)/negative arm A/CELL 8 ==
  mod : Inport
  DC Voltage Source : fl_lib/Electrical/Electrical Sources/DC Voltage Source  v0=Vcell V
  Ideal Half-Bridge : ee_lib_for_power_systems/Power Converters/Ideal Half-Bridge  Vf=0.5  Ron=Ron  Goff=Goff  run_time=off
      settings: SourceProductName=Support Library for Power Systems
  + : PMIOPort  Side=Left
  - : PMIOPort  Port=2  Side=Left
  wires:
  mod/1 -> Ideal Half-Bridge/1
  connections:
  -/RConn1 -- DC Voltage Source/RConn1 -- Ideal Half-Bridge/RConn2
  Ideal Half-Bridge/RConn1 -- DC Voltage Source/LConn1
  Ideal Half-Bridge/LConn1 -- +/RConn1

== system MMC_driven_PMSM_ideal/MMC 8 Cell (Ideal)/negative arm B/CELL 1 ==
  mod : Inport
  DC Voltage Source : fl_lib/Electrical/Electrical Sources/DC Voltage Source  v0=Vcell V
  Ideal Half-Bridge : ee_lib_for_power_systems/Power Converters/Ideal Half-Bridge  Vf=0.5  Ron=Ron  Goff=Goff  run_time=off
      settings: SourceProductName=Support Library for Power Systems
  + : PMIOPort  Side=Left
  - : PMIOPort  Port=2  Side=Left
  wires:
  mod/1 -> Ideal Half-Bridge/1
  connections:
  -/RConn1 -- DC Voltage Source/RConn1 -- Ideal Half-Bridge/RConn2
  Ideal Half-Bridge/RConn1 -- DC Voltage Source/LConn1
  Ideal Half-Bridge/LConn1 -- +/RConn1

== system MMC_driven_PMSM_ideal/MMC 8 Cell (Ideal)/negative arm B/CELL 2 ==
  mod : Inport
  DC Voltage Source : fl_lib/Electrical/Electrical Sources/DC Voltage Source  v0=Vcell V
  Ideal Half-Bridge : ee_lib_for_power_systems/Power Converters/Ideal Half-Bridge  Vf=0.5  Ron=Ron  Goff=Goff  run_time=off
      settings: SourceProductName=Support Library for Power Systems
  + : PMIOPort  Side=Left
  - : PMIOPort  Port=2  Side=Left
  wires:
  mod/1 -> Ideal Half-Bridge/1
  connections:
  Ideal Half-Bridge/LConn1 -- +/RConn1
  Ideal Half-Bridge/RConn1 -- DC Voltage Source/LConn1
  Ideal Half-Bridge/RConn2 -- DC Voltage Source/RConn1 -- -/RConn1

== system MMC_driven_PMSM_ideal/MMC 8 Cell (Ideal)/negative arm B/CELL 3 ==
  mod : Inport
  DC Voltage Source : fl_lib/Electrical/Electrical Sources/DC Voltage Source  v0=Vcell V
  Ideal Half-Bridge : ee_lib_for_power_systems/Power Converters/Ideal Half-Bridge  Vf=0.5  Ron=Ron  Goff=Goff  run_time=off
      settings: SourceProductName=Support Library for Power Systems
  + : PMIOPort  Side=Left
  - : PMIOPort  Port=2  Side=Left
  wires:
  mod/1 -> Ideal Half-Bridge/1
  connections:
  -/RConn1 -- DC Voltage Source/RConn1 -- Ideal Half-Bridge/RConn2
  Ideal Half-Bridge/RConn1 -- DC Voltage Source/LConn1
  Ideal Half-Bridge/LConn1 -- +/RConn1

== system MMC_driven_PMSM_ideal/MMC 8 Cell (Ideal)/negative arm B/CELL 4 ==
  mod : Inport
  DC Voltage Source : fl_lib/Electrical/Electrical Sources/DC Voltage Source  v0=Vcell V
  Ideal Half-Bridge : ee_lib_for_power_systems/Power Converters/Ideal Half-Bridge  Vf=0.5  Ron=Ron  Goff=Goff  run_time=off
      settings: SourceProductName=Support Library for Power Systems
  + : PMIOPort  Side=Left
  - : PMIOPort  Port=2  Side=Left
  wires:
  mod/1 -> Ideal Half-Bridge/1
  connections:
  Ideal Half-Bridge/LConn1 -- +/RConn1
  Ideal Half-Bridge/RConn1 -- DC Voltage Source/LConn1
  Ideal Half-Bridge/RConn2 -- DC Voltage Source/RConn1 -- -/RConn1

== system MMC_driven_PMSM_ideal/MMC 8 Cell (Ideal)/negative arm B/CELL 5 ==
  mod : Inport
  DC Voltage Source : fl_lib/Electrical/Electrical Sources/DC Voltage Source  v0=Vcell V
  Ideal Half-Bridge : ee_lib_for_power_systems/Power Converters/Ideal Half-Bridge  Vf=0.5  Ron=Ron  Goff=Goff  run_time=off
      settings: SourceProductName=Support Library for Power Systems
  + : PMIOPort  Side=Left
  - : PMIOPort  Port=2  Side=Left
  wires:
  mod/1 -> Ideal Half-Bridge/1
  connections:
  -/RConn1 -- DC Voltage Source/RConn1 -- Ideal Half-Bridge/RConn2
  Ideal Half-Bridge/RConn1 -- DC Voltage Source/LConn1
  Ideal Half-Bridge/LConn1 -- +/RConn1

== system MMC_driven_PMSM_ideal/MMC 8 Cell (Ideal)/negative arm B/CELL 6 ==
  mod : Inport
  DC Voltage Source : fl_lib/Electrical/Electrical Sources/DC Voltage Source  v0=Vcell V
  Ideal Half-Bridge : ee_lib_for_power_systems/Power Converters/Ideal Half-Bridge  Vf=0.5  Ron=Ron  Goff=Goff  run_time=off
      settings: SourceProductName=Support Library for Power Systems
  + : PMIOPort  Side=Left
  - : PMIOPort  Port=2  Side=Left
  wires:
  mod/1 -> Ideal Half-Bridge/1
  connections:
  Ideal Half-Bridge/LConn1 -- +/RConn1
  Ideal Half-Bridge/RConn1 -- DC Voltage Source/LConn1
  Ideal Half-Bridge/RConn2 -- DC Voltage Source/RConn1 -- -/RConn1

== system MMC_driven_PMSM_ideal/MMC 8 Cell (Ideal)/negative arm B/CELL 7 ==
  mod : Inport
  DC Voltage Source : fl_lib/Electrical/Electrical Sources/DC Voltage Source  v0=Vcell V
  Ideal Half-Bridge : ee_lib_for_power_systems/Power Converters/Ideal Half-Bridge  Vf=0.5  Ron=Ron  Goff=Goff  run_time=off
      settings: SourceProductName=Support Library for Power Systems
  + : PMIOPort  Side=Left
  - : PMIOPort  Port=2  Side=Left
  wires:
  mod/1 -> Ideal Half-Bridge/1
  connections:
  -/RConn1 -- DC Voltage Source/RConn1 -- Ideal Half-Bridge/RConn2
  Ideal Half-Bridge/RConn1 -- DC Voltage Source/LConn1
  Ideal Half-Bridge/LConn1 -- +/RConn1

== system MMC_driven_PMSM_ideal/MMC 8 Cell (Ideal)/negative arm B/CELL 8 ==
  mod : Inport
  DC Voltage Source : fl_lib/Electrical/Electrical Sources/DC Voltage Source  v0=Vcell V
  Ideal Half-Bridge : ee_lib_for_power_systems/Power Converters/Ideal Half-Bridge  Vf=0.5  Ron=Ron  Goff=Goff  run_time=off
      settings: SourceProductName=Support Library for Power Systems
  + : PMIOPort  Side=Left
  - : PMIOPort  Port=2  Side=Left
  wires:
  mod/1 -> Ideal Half-Bridge/1
  connections:
  Ideal Half-Bridge/LConn1 -- +/RConn1
  Ideal Half-Bridge/RConn1 -- DC Voltage Source/LConn1
  Ideal Half-Bridge/RConn2 -- DC Voltage Source/RConn1 -- -/RConn1

== system MMC_driven_PMSM_ideal/MMC 8 Cell (Ideal)/negative arm C/CELL 1 ==
  mod : Inport
  DC Voltage Source : fl_lib/Electrical/Electrical Sources/DC Voltage Source  v0=Vcell V
  Ideal Half-Bridge : ee_lib_for_power_systems/Power Converters/Ideal Half-Bridge  Vf=0.5  Ron=Ron  Goff=Goff  run_time=off
      settings: SourceProductName=Support Library for Power Systems
  + : PMIOPort  Side=Left
  - : PMIOPort  Port=2  Side=Left
  wires:
  mod/1 -> Ideal Half-Bridge/1
  connections:
  Ideal Half-Bridge/LConn1 -- +/RConn1
  Ideal Half-Bridge/RConn1 -- DC Voltage Source/LConn1
  Ideal Half-Bridge/RConn2 -- DC Voltage Source/RConn1 -- -/RConn1

== system MMC_driven_PMSM_ideal/MMC 8 Cell (Ideal)/negative arm C/CELL 2 ==
  mod : Inport
  DC Voltage Source : fl_lib/Electrical/Electrical Sources/DC Voltage Source  v0=Vcell V
  Ideal Half-Bridge : ee_lib_for_power_systems/Power Converters/Ideal Half-Bridge  Vf=0.5  Ron=Ron  Goff=Goff  run_time=off
      settings: SourceProductName=Support Library for Power Systems
  + : PMIOPort  Side=Left
  - : PMIOPort  Port=2  Side=Left
  wires:
  mod/1 -> Ideal Half-Bridge/1
  connections:
  -/RConn1 -- DC Voltage Source/RConn1 -- Ideal Half-Bridge/RConn2
  Ideal Half-Bridge/RConn1 -- DC Voltage Source/LConn1
  Ideal Half-Bridge/LConn1 -- +/RConn1

== system MMC_driven_PMSM_ideal/MMC 8 Cell (Ideal)/negative arm C/CELL 3 ==
  mod : Inport
  DC Voltage Source : fl_lib/Electrical/Electrical Sources/DC Voltage Source  v0=Vcell V
  Ideal Half-Bridge : ee_lib_for_power_systems/Power Converters/Ideal Half-Bridge  Vf=0.5  Ron=Ron  Goff=Goff  run_time=off
      settings: SourceProductName=Support Library for Power Systems
  + : PMIOPort  Side=Left
  - : PMIOPort  Port=2  Side=Left
  wires:
  mod/1 -> Ideal Half-Bridge/1
  connections:
  Ideal Half-Bridge/LConn1 -- +/RConn1
  Ideal Half-Bridge/RConn1 -- DC Voltage Source/LConn1
  Ideal Half-Bridge/RConn2 -- DC Voltage Source/RConn1 -- -/RConn1

== system MMC_driven_PMSM_ideal/MMC 8 Cell (Ideal)/negative arm C/CELL 4 ==
  mod : Inport
  DC Voltage Source : fl_lib/Electrical/Electrical Sources/DC Voltage Source  v0=Vcell V
  Ideal Half-Bridge : ee_lib_for_power_systems/Power Converters/Ideal Half-Bridge  Vf=0.5  Ron=Ron  Goff=Goff  run_time=off
      settings: SourceProductName=Support Library for Power Systems
  + : PMIOPort  Side=Left
  - : PMIOPort  Port=2  Side=Left
  wires:
  mod/1 -> Ideal Half-Bridge/1
  connections:
  -/RConn1 -- DC Voltage Source/RConn1 -- Ideal Half-Bridge/RConn2
  Ideal Half-Bridge/RConn1 -- DC Voltage Source/LConn1
  Ideal Half-Bridge/LConn1 -- +/RConn1

== system MMC_driven_PMSM_ideal/MMC 8 Cell (Ideal)/negative arm C/CELL 5 ==
  mod : Inport
  DC Voltage Source : fl_lib/Electrical/Electrical Sources/DC Voltage Source  v0=Vcell V
  Ideal Half-Bridge : ee_lib_for_power_systems/Power Converters/Ideal Half-Bridge  Vf=0.5  Ron=Ron  Goff=Goff  run_time=off
      settings: SourceProductName=Support Library for Power Systems
  + : PMIOPort  Side=Left
  - : PMIOPort  Port=2  Side=Left
  wires:
  mod/1 -> Ideal Half-Bridge/1
  connections:
  Ideal Half-Bridge/LConn1 -- +/RConn1
  Ideal Half-Bridge/RConn1 -- DC Voltage Source/LConn1
  Ideal Half-Bridge/RConn2 -- DC Voltage Source/RConn1 -- -/RConn1

== system MMC_driven_PMSM_ideal/MMC 8 Cell (Ideal)/negative arm C/CELL 6 ==
  mod : Inport
  DC Voltage Source : fl_lib/Electrical/Electrical Sources/DC Voltage Source  v0=Vcell V
  Ideal Half-Bridge : ee_lib_for_power_systems/Power Converters/Ideal Half-Bridge  Vf=0.5  Ron=Ron  Goff=Goff  run_time=off
      settings: SourceProductName=Support Library for Power Systems
  + : PMIOPort  Side=Left
  - : PMIOPort  Port=2  Side=Left
  wires:
  mod/1 -> Ideal Half-Bridge/1
  connections:
  -/RConn1 -- DC Voltage Source/RConn1 -- Ideal Half-Bridge/RConn2
  Ideal Half-Bridge/RConn1 -- DC Voltage Source/LConn1
  Ideal Half-Bridge/LConn1 -- +/RConn1

== system MMC_driven_PMSM_ideal/MMC 8 Cell (Ideal)/negative arm C/CELL 7 ==
  mod : Inport
  DC Voltage Source : fl_lib/Electrical/Electrical Sources/DC Voltage Source  v0=Vcell V
  Ideal Half-Bridge : ee_lib_for_power_systems/Power Converters/Ideal Half-Bridge  Vf=0.5  Ron=Ron  Goff=Goff  run_time=off
      settings: SourceProductName=Support Library for Power Systems
  + : PMIOPort  Side=Left
  - : PMIOPort  Port=2  Side=Left
  wires:
  mod/1 -> Ideal Half-Bridge/1
  connections:
  Ideal Half-Bridge/LConn1 -- +/RConn1
  Ideal Half-Bridge/RConn1 -- DC Voltage Source/LConn1
  Ideal Half-Bridge/RConn2 -- DC Voltage Source/RConn1 -- -/RConn1

== system MMC_driven_PMSM_ideal/MMC 8 Cell (Ideal)/negative arm C/CELL 8 ==
  mod : Inport
  DC Voltage Source : fl_lib/Electrical/Electrical Sources/DC Voltage Source  v0=Vcell V
  Ideal Half-Bridge : ee_lib_for_power_systems/Power Converters/Ideal Half-Bridge  Vf=0.5  Ron=Ron  Goff=Goff  run_time=off
      settings: SourceProductName=Support Library for Power Systems
  + : PMIOPort  Side=Left
  - : PMIOPort  Port=2  Side=Left
  wires:
  mod/1 -> Ideal Half-Bridge/1
  connections:
  -/RConn1 -- DC Voltage Source/RConn1 -- Ideal Half-Bridge/RConn2
  Ideal Half-Bridge/RConn1 -- DC Voltage Source/LConn1
  Ideal Half-Bridge/LConn1 -- +/RConn1

== system MMC_driven_PMSM_ideal/MMC 8 Cell (Ideal)/positive arm A/CELL 1 ==
  mod : Inport
  DC Voltage Source : fl_lib/Electrical/Electrical Sources/DC Voltage Source  v0=Vcell V
  Ideal Half-Bridge : ee_lib_for_power_systems/Power Converters/Ideal Half-Bridge  Vf=0.5  Ron=Ron  Goff=Goff  run_time=off
      settings: SourceProductName=Support Library for Power Systems
  + : PMIOPort  Side=Left
  - : PMIOPort  Port=2  Side=Left
  wires:
  mod/1 -> Ideal Half-Bridge/1
  connections:
  -/RConn1 -- Ideal Half-Bridge/RConn2 -- DC Voltage Source/RConn1
  Ideal Half-Bridge/RConn1 -- DC Voltage Source/LConn1
  Ideal Half-Bridge/LConn1 -- +/RConn1

== system MMC_driven_PMSM_ideal/MMC 8 Cell (Ideal)/positive arm A/CELL 2 ==
  mod : Inport
  DC Voltage Source : fl_lib/Electrical/Electrical Sources/DC Voltage Source  v0=Vcell V
  Ideal Half-Bridge : ee_lib_for_power_systems/Power Converters/Ideal Half-Bridge  Vf=0.5  Ron=Ron  Goff=Goff  run_time=off
      settings: SourceProductName=Support Library for Power Systems
  + : PMIOPort  Side=Left
  - : PMIOPort  Port=2  Side=Left
  wires:
  mod/1 -> Ideal Half-Bridge/1
  connections:
  Ideal Half-Bridge/LConn1 -- +/RConn1
  Ideal Half-Bridge/RConn1 -- DC Voltage Source/LConn1
  Ideal Half-Bridge/RConn2 -- DC Voltage Source/RConn1 -- -/RConn1

== system MMC_driven_PMSM_ideal/MMC 8 Cell (Ideal)/positive arm A/CELL 3 ==
  mod : Inport
  DC Voltage Source : fl_lib/Electrical/Electrical Sources/DC Voltage Source  v0=Vcell V
  Ideal Half-Bridge : ee_lib_for_power_systems/Power Converters/Ideal Half-Bridge  Vf=0.5  Ron=Ron  Goff=Goff  run_time=off
      settings: SourceProductName=Support Library for Power Systems
  + : PMIOPort  Side=Left
  - : PMIOPort  Port=2  Side=Left
  wires:
  mod/1 -> Ideal Half-Bridge/1
  connections:
  -/RConn1 -- DC Voltage Source/RConn1 -- Ideal Half-Bridge/RConn2
  Ideal Half-Bridge/RConn1 -- DC Voltage Source/LConn1
  Ideal Half-Bridge/LConn1 -- +/RConn1

== system MMC_driven_PMSM_ideal/MMC 8 Cell (Ideal)/positive arm A/CELL 4 ==
  mod : Inport
  DC Voltage Source : fl_lib/Electrical/Electrical Sources/DC Voltage Source  v0=Vcell V
  Ideal Half-Bridge : ee_lib_for_power_systems/Power Converters/Ideal Half-Bridge  Vf=0.5  Ron=Ron  Goff=Goff  run_time=off
      settings: SourceProductName=Support Library for Power Systems
  + : PMIOPort  Side=Left
  - : PMIOPort  Port=2  Side=Left
  wires:
  mod/1 -> Ideal Half-Bridge/1
  connections:
  Ideal Half-Bridge/LConn1 -- +/RConn1
  Ideal Half-Bridge/RConn1 -- DC Voltage Source/LConn1
  Ideal Half-Bridge/RConn2 -- DC Voltage Source/RConn1 -- -/RConn1

== system MMC_driven_PMSM_ideal/MMC 8 Cell (Ideal)/positive arm A/CELL 5 ==
  mod : Inport
  DC Voltage Source : fl_lib/Electrical/Electrical Sources/DC Voltage Source  v0=Vcell V
  Ideal Half-Bridge : ee_lib_for_power_systems/Power Converters/Ideal Half-Bridge  Vf=0.5  Ron=Ron  Goff=Goff  run_time=off
      settings: SourceProductName=Support Library for Power Systems
  + : PMIOPort  Side=Left
  - : PMIOPort  Port=2  Side=Left
  wires:
  mod/1 -> Ideal Half-Bridge/1
  connections:
  -/RConn1 -- DC Voltage Source/RConn1 -- Ideal Half-Bridge/RConn2
  Ideal Half-Bridge/RConn1 -- DC Voltage Source/LConn1
  Ideal Half-Bridge/LConn1 -- +/RConn1

== system MMC_driven_PMSM_ideal/MMC 8 Cell (Ideal)/positive arm A/CELL 6 ==
  mod : Inport
  DC Voltage Source : fl_lib/Electrical/Electrical Sources/DC Voltage Source  v0=Vcell V
  Ideal Half-Bridge : ee_lib_for_power_systems/Power Converters/Ideal Half-Bridge  Vf=0.5  Ron=Ron  Goff=Goff  run_time=off
      settings: SourceProductName=Support Library for Power Systems
  + : PMIOPort  Side=Left
  - : PMIOPort  Port=2  Side=Left
  wires:
  mod/1 -> Ideal Half-Bridge/1
  connections:
  Ideal Half-Bridge/LConn1 -- +/RConn1
  Ideal Half-Bridge/RConn1 -- DC Voltage Source/LConn1
  Ideal Half-Bridge/RConn2 -- DC Voltage Source/RConn1 -- -/RConn1

== system MMC_driven_PMSM_ideal/MMC 8 Cell (Ideal)/positive arm A/CELL 7 ==
  mod : Inport
  DC Voltage Source : fl_lib/Electrical/Electrical Sources/DC Voltage Source  v0=Vcell V
  Ideal Half-Bridge : ee_lib_for_power_systems/Power Converters/Ideal Half-Bridge  Vf=0.5  Ron=Ron  Goff=Goff  run_time=off
      settings: SourceProductName=Support Library for Power Systems
  + : PMIOPort  Side=Left
  - : PMIOPort  Port=2  Side=Left
  wires:
  mod/1 -> Ideal Half-Bridge/1
  connections:
  -/RConn1 -- DC Voltage Source/RConn1 -- Ideal Half-Bridge/RConn2
  Ideal Half-Bridge/RConn1 -- DC Voltage Source/LConn1
  Ideal Half-Bridge/LConn1 -- +/RConn1

== system MMC_driven_PMSM_ideal/MMC 8 Cell (Ideal)/positive arm A/CELL 8 ==
  mod : Inport
  DC Voltage Source : fl_lib/Electrical/Electrical Sources/DC Voltage Source  v0=Vcell V
  Ideal Half-Bridge : ee_lib_for_power_systems/Power Converters/Ideal Half-Bridge  Vf=0.5  Ron=Ron  Goff=Goff  run_time=off
      settings: SourceProductName=Support Library for Power Systems
  + : PMIOPort  Side=Left
  - : PMIOPort  Port=2  Side=Left
  wires:
  mod/1 -> Ideal Half-Bridge/1
  connections:
  Ideal Half-Bridge/LConn1 -- +/RConn1
  Ideal Half-Bridge/RConn1 -- DC Voltage Source/LConn1
  Ideal Half-Bridge/RConn2 -- DC Voltage Source/RConn1 -- -/RConn1

== system MMC_driven_PMSM_ideal/MMC 8 Cell (Ideal)/positive arm B/CELL 1 ==
  mod : Inport
  DC Voltage Source : fl_lib/Electrical/Electrical Sources/DC Voltage Source  v0=Vcell V
  Ideal Half-Bridge : ee_lib_for_power_systems/Power Converters/Ideal Half-Bridge  Vf=0.5  Ron=Ron  Goff=Goff  run_time=off
      settings: SourceProductName=Support Library for Power Systems
  + : PMIOPort  Side=Left
  - : PMIOPort  Port=2  Side=Left
  wires:
  mod/1 -> Ideal Half-Bridge/1
  connections:
  Ideal Half-Bridge/LConn1 -- +/RConn1
  Ideal Half-Bridge/RConn1 -- DC Voltage Source/LConn1
  Ideal Half-Bridge/RConn2 -- DC Voltage Source/RConn1 -- -/RConn1

== system MMC_driven_PMSM_ideal/MMC 8 Cell (Ideal)/positive arm B/CELL 2 ==
  mod : Inport
  DC Voltage Source : fl_lib/Electrical/Electrical Sources/DC Voltage Source  v0=Vcell V
  Ideal Half-Bridge : ee_lib_for_power_systems/Power Converters/Ideal Half-Bridge  Vf=0.5  Ron=Ron  Goff=Goff  run_time=off
      settings: SourceProductName=Support Library for Power Systems
  + : PMIOPort  Side=Left
  - : PMIOPort  Port=2  Side=Left
  wires:
  mod/1 -> Ideal Half-Bridge/1
  connections:
  -/RConn1 -- DC Voltage Source/RConn1 -- Ideal Half-Bridge/RConn2
  Ideal Half-Bridge/RConn1 -- DC Voltage Source/LConn1
  Ideal Half-Bridge/LConn1 -- +/RConn1

== system MMC_driven_PMSM_ideal/MMC 8 Cell (Ideal)/positive arm B/CELL 3 ==
  mod : Inport
  DC Voltage Source : fl_lib/Electrical/Electrical Sources/DC Voltage Source  v0=Vcell V
  Ideal Half-Bridge : ee_lib_for_power_systems/Power Converters/Ideal Half-Bridge  Vf=0.5  Ron=Ron  Goff=Goff  run_time=off
      settings: SourceProductName=Support Library for Power Systems
  + : PMIOPort  Side=Left
  - : PMIOPort  Port=2  Side=Left
  wires:
  mod/1 -> Ideal Half-Bridge/1
  connections:
  Ideal Half-Bridge/LConn1 -- +/RConn1
  Ideal Half-Bridge/RConn1 -- DC Voltage Source/LConn1
  Ideal Half-Bridge/RConn2 -- DC Voltage Source/RConn1 -- -/RConn1

== system MMC_driven_PMSM_ideal/MMC 8 Cell (Ideal)/positive arm B/CELL 4 ==
  mod : Inport
  DC Voltage Source : fl_lib/Electrical/Electrical Sources/DC Voltage Source  v0=Vcell V
  Ideal Half-Bridge : ee_lib_for_power_systems/Power Converters/Ideal Half-Bridge  Vf=0.5  Ron=Ron  Goff=Goff  run_time=off
      settings: SourceProductName=Support Library for Power Systems
  + : PMIOPort  Side=Left
  - : PMIOPort  Port=2  Side=Left
  wires:
  mod/1 -> Ideal Half-Bridge/1
  connections:
  -/RConn1 -- DC Voltage Source/RConn1 -- Ideal Half-Bridge/RConn2
  Ideal Half-Bridge/RConn1 -- DC Voltage Source/LConn1
  Ideal Half-Bridge/LConn1 -- +/RConn1

== system MMC_driven_PMSM_ideal/MMC 8 Cell (Ideal)/positive arm B/CELL 5 ==
  mod : Inport
  DC Voltage Source : fl_lib/Electrical/Electrical Sources/DC Voltage Source  v0=Vcell V
  Ideal Half-Bridge : ee_lib_for_power_systems/Power Converters/Ideal Half-Bridge  Vf=0.5  Ron=Ron  Goff=Goff  run_time=off
      settings: SourceProductName=Support Library for Power Systems
  + : PMIOPort  Side=Left
  - : PMIOPort  Port=2  Side=Left
  wires:
  mod/1 -> Ideal Half-Bridge/1
  connections:
  Ideal Half-Bridge/LConn1 -- +/RConn1
  Ideal Half-Bridge/RConn1 -- DC Voltage Source/LConn1
  Ideal Half-Bridge/RConn2 -- DC Voltage Source/RConn1 -- -/RConn1

== system MMC_driven_PMSM_ideal/MMC 8 Cell (Ideal)/positive arm B/CELL 6 ==
  mod : Inport
  DC Voltage Source : fl_lib/Electrical/Electrical Sources/DC Voltage Source  v0=Vcell V
  Ideal Half-Bridge : ee_lib_for_power_systems/Power Converters/Ideal Half-Bridge  Vf=0.5  Ron=Ron  Goff=Goff  run_time=off
      settings: SourceProductName=Support Library for Power Systems
  + : PMIOPort  Side=Left
  - : PMIOPort  Port=2  Side=Left
  wires:
  mod/1 -> Ideal Half-Bridge/1
  connections:
  -/RConn1 -- DC Voltage Source/RConn1 -- Ideal Half-Bridge/RConn2
  Ideal Half-Bridge/RConn1 -- DC Voltage Source/LConn1
  Ideal Half-Bridge/LConn1 -- +/RConn1
